simulink model "sampleModel1888"  (R2023a)
settings: Solver=VariableStepAuto  StartTime=0.0  StopTime=10.0  RelTol=1e-3
libraries: hdlsllib x4, simulink x3
settings Model: Creator=user1  LastModifiedBy=user1

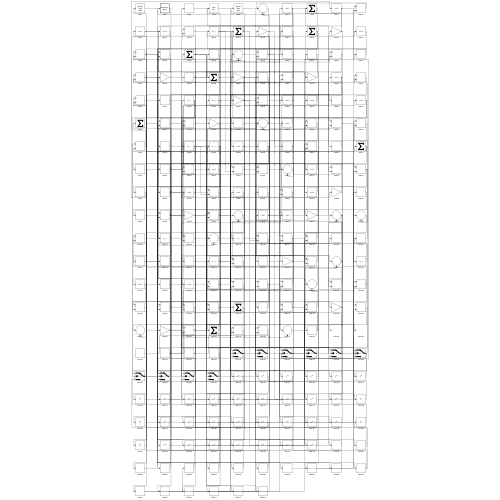
[thumbnail: Simulink's stored preview of the top-level diagram]
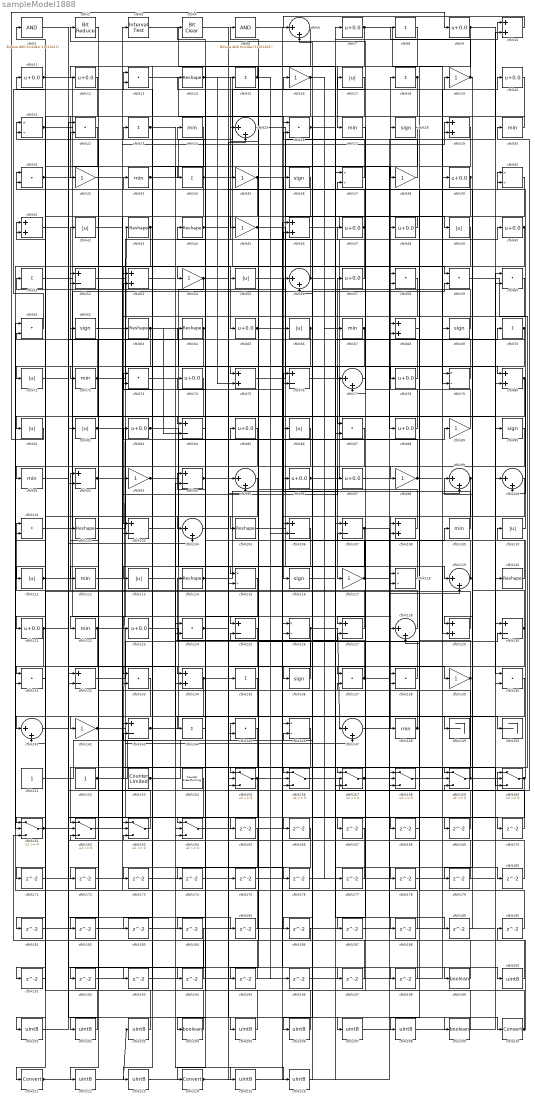
== system sampleModel1888 ==
  cfblk1 : simulink/Logic and Bit Operations/Bitwise Operator  logicop=AND  UseBitMask=on  BitMask=bin2dec('11011001')  BitMaskRealWorld=Stored Integer
      settings: LibrarySourceBlock=|
      | hdlsllib/Logic and Bit
      | Operations/Bitwise
      | Operator
  cfblk{10,29,41,46,53,68,75,80,108,129,134} (11 alike) : Sum
  cfblk{6,25,56,77,95,99..100,104,119,128,141,147} (12 alike) : Sum  Inputs=|++
  cfblk{13,22,26,31,58..61,73,87,101,124,131,133,137..138,140,145} (18 alike) : DotProduct  OutDataTypeStr=Inherit: Inherit via internal rule
  cfblk{14,43..44,63..64,102,105,114,120} (9 alike) : Reshape
  cfblk{52,76,84,92,94,103,106..107,125,127,130,132,143} (13 alike) : Sum  Inputs=+-
  cfblk{24,27,30,33,67,72,91,109,112,122,148} (11 alike) : MinMax
  cfblk{7,9,11..12,20,39,47..48,50,57,65,74,78,83,85,88,96..97,121,123} (20 alike) : Bias  Bias=0.0  SaturateOnIntegerOverflow=off
  cfblk{17,42,49,55,66,71,81..82,86,110..111,113} (12 alike) : Abs  SaturateOnIntegerOverflow=off
  cfblk{21,37,40,79,115,118,126,146} (8 alike) : Product  Inputs=*/  RndMeth=Zero  SaturateOnIntegerOverflow=on
  cfblk{28,36,62,69,90,116,136} (7 alike) : Signum
  cfblk{16,19,32,35,38,45,54,89,93,98,117,139,142} (13 alike) : Gain
  cfblk{8,15,18,23,34,51,70,135,144} (9 alike) : Sum  Inputs=+
  cfblk149 : Terminator
  cfblk150 : Terminator
  cfblk151 : Constant  SampleTime=-1
  cfblk152 : Constant  SampleTime=-1
  cfblk153 : hdlsllib/Sources/Counter Limited  uplimit=7  tsamp=-1
  cfblk154 : hdlsllib/Sources/Counter Free-Running  NumBits=16  tsamp=-1
  cfblk{155..164} (10 alike) : Switch  SaturateOnIntegerOverflow=off  InputSameDT=off
  cfblk{165..198} (34 alike) : Delay  SampleTime=1
  cfblk199 : DataTypeConversion  OutDataTypeStr=boolean  SaturateOnIntegerOverflow=off  RndMeth=Floor
  cfblk2 : hdlsllib/Logic and Bit Operations/Bit Reduce  mode=AND
  cfblk{200..203,205..208,212..213,215..216} (12 alike) : DataTypeConversion  OutDataTypeStr=uint8  SaturateOnIntegerOverflow=off  RndMeth=Floor
  cfblk204 : DataTypeConversion  OutDataTypeStr=boolean  SaturateOnIntegerOverflow=off  RndMeth=Floor
  cfblk209 : DataTypeConversion  OutDataTypeStr=boolean  SaturateOnIntegerOverflow=off  RndMeth=Floor
  cfblk210 : DataTypeConversion  SaturateOnIntegerOverflow=off  RndMeth=Floor
  cfblk211 : DataTypeConversion  SaturateOnIntegerOverflow=off  RndMeth=Floor
  cfblk214 : DataTypeConversion  SaturateOnIntegerOverflow=off  RndMeth=Floor
  cfblk3 : hdlsllib/Logic and Bit Operations/Interval Test  IntervalClosedRight=on  uplimit=0.5  IntervalClosedLeft=on  lowlimit=-0.5  OutDataTypeStr=boolean
  cfblk4 : simulink/Logic and Bit Operations/Bit Clear  iBit=0
      settings: LibrarySourceBlock=|
      | hdlsllib/Logic and Bit
      | Operations/Bit Clear
  cfblk5 : simulink/Logic and Bit Operations/Bitwise Operator  logicop=AND  UseBitMask=on  BitMask=bin2dec('11011001')  BitMaskRealWorld=Stored Integer
      settings: LibrarySourceBlock=|
      | hdlsllib/Logic and Bit
      | Operations/Bitwise
      | Operator
  wires:
  cfblk122/1 -> cfblk164/1, cfblk131/1
  cfblk75/1 -> cfblk40/1
  cfblk153/1 -> cfblk51/1, cfblk86/1
  cfblk80/1 -> cfblk100/2, cfblk212/1
  cfblk70/1 -> cfblk61/2, cfblk187/1
  cfblk59/1 -> cfblk156/1
  cfblk160/1 -> cfblk110/1, cfblk186/1
  cfblk14/1 -> cfblk59/1, cfblk75/2, cfblk159/2
  cfblk99/1 -> cfblk148/1, cfblk149/1
  cfblk31/1 -> cfblk65/1, cfblk133/2
  cfblk46/1 -> cfblk49/1
  cfblk21/1 -> cfblk125/1, cfblk193/1
  cfblk118/1 -> cfblk24/1
  cfblk132/1 -> cfblk130/2
  cfblk16/1 -> cfblk54/1, cfblk67/1
  cfblk13/1 -> cfblk116/1
  cfblk88/1 -> cfblk18/1
  cfblk155/1 -> cfblk109/1, cfblk183/1
  cfblk152/1 -> cfblk43/1, cfblk94/2
  cfblk146/1 -> cfblk214/1
  cfblk102/1 -> cfblk39/1
  cfblk161/1 -> cfblk160/1, cfblk185/1
  cfblk8/1 -> cfblk27/1
  cfblk19/1 -> cfblk129/1, cfblk8/1
  cfblk45/1 -> cfblk118/1, cfblk106/2
  cfblk143/1 -> cfblk47/1, cfblk127/2
  cfblk136/1 -> cfblk114/1
  cfblk164/1 -> cfblk46/1
  cfblk57/1 -> cfblk55/1
  cfblk79/1 -> cfblk42/1
  cfblk90/1 -> cfblk117/1
  cfblk63/1 -> cfblk75/1, cfblk72/1, cfblk84/2, cfblk160/3
  cfblk96/1 -> cfblk50/1, cfblk46/2, cfblk70/1
  cfblk159/1 -> cfblk90/1, cfblk137/2
  cfblk109/1 -> cfblk76/1
  cfblk82/1 -> cfblk128/1, cfblk29/2, cfblk134/2
  cfblk26/1 -> cfblk177/1, cfblk178/1
  cfblk72/1 -> cfblk15/1, cfblk77/1, cfblk41/2, cfblk111/1
  cfblk55/1 -> cfblk78/1
  cfblk74/1 -> cfblk81/1
  cfblk101/1 -> cfblk58/1
  cfblk113/1 -> cfblk157/1
  cfblk9/1 -> cfblk140/1, cfblk208/1
  cfblk43/1 -> cfblk103/1, cfblk103/2, cfblk131/2
  cfblk156/1 -> cfblk30/1
  cfblk85/1 -> cfblk93/1
  cfblk17/1 -> cfblk136/1
  cfblk97/1 -> cfblk68/1
  cfblk145/1 -> cfblk162/1
  cfblk83/1 -> cfblk118/2, cfblk23/1
  cfblk111/1 -> cfblk123/1, cfblk104/2
  cfblk18/1 -> cfblk32/1, cfblk121/1
  cfblk61/1 -> cfblk13/1
  cfblk87/1 -> cfblk91/1
  cfblk69/1 -> cfblk14/1
  cfblk36/1 -> cfblk122/1
  cfblk123/1 -> cfblk125/2
  cfblk58/1 -> cfblk113/1
  cfblk73/1 -> cfblk56/1
  cfblk114/1 -> cfblk57/1, cfblk139/1
  cfblk29/1 -> cfblk98/1
  cfblk54/1 -> cfblk53/2, cfblk170/1
  cfblk86/1 -> cfblk115/1
  cfblk56/1 -> cfblk10/1, cfblk35/1
  cfblk3/1 -> cfblk107/1
  cfblk128/1 -> cfblk101/1
  cfblk51/1 -> cfblk87/1
  cfblk124/1 -> cfblk44/1, cfblk37/2, cfblk194/1
  cfblk66/1 -> cfblk126/2, cfblk191/1
  cfblk89/1 -> cfblk2/1
  cfblk48/1 -> cfblk45/1
  cfblk120/1 -> cfblk74/1
  cfblk81/1 -> cfblk9/1
  cfblk110/1 -> cfblk40/2
  cfblk117/1 -> cfblk48/1, cfblk36/1
  cfblk154/1 -> cfblk162/2
  cfblk93/1 -> cfblk89/1, cfblk159/1
  cfblk44/1 -> cfblk134/1, cfblk166/1
  cfblk126/1 -> cfblk147/1, cfblk171/1
  cfblk33/1 -> cfblk19/1, cfblk38/1
  cfblk121/1 -> cfblk64/1, cfblk161/2
  cfblk112/1 -> cfblk155/1
  cfblk95/1 -> cfblk211/1
  cfblk30/1 -> cfblk26/1
  cfblk84/1 -> cfblk144/1
  cfblk127/1 -> cfblk92/1
  cfblk158/1 -> cfblk99/2
  cfblk139/1 -> cfblk31/1, cfblk156/3
  cfblk142/1 -> cfblk147/2, cfblk168/1
  cfblk140/1 -> cfblk143/1
  cfblk40/1 -> cfblk155/2
  cfblk28/1 -> cfblk156/2
  cfblk32/1 -> cfblk3/1
  cfblk77/1 -> cfblk127/1
  cfblk50/1 -> cfblk141/1, cfblk77/2
  cfblk98/1 -> cfblk20/1, cfblk13/2
  cfblk67/1 -> cfblk161/1, cfblk17/1
  cfblk92/1 -> cfblk76/2, cfblk164/3, cfblk160/2
  cfblk42/1 -> cfblk80/1
  cfblk108/1 -> cfblk25/1
  cfblk38/1 -> cfblk28/1
  cfblk49/1 -> cfblk104/1
  cfblk131/1 -> cfblk141/2
  cfblk137/1 -> cfblk96/1, cfblk189/1
  cfblk35/1 -> cfblk10/2, cfblk71/1, cfblk197/1
  cfblk27/1 -> cfblk137/1
  cfblk148/1 -> cfblk73/1, cfblk102/1
  cfblk135/1 -> cfblk164/2
  cfblk37/1 -> cfblk16/1
  cfblk68/1 -> cfblk108/1
  cfblk39/1 -> cfblk112/1, cfblk124/2
  cfblk78/1 -> cfblk41/1
  cfblk100/1 -> cfblk106/1
  cfblk20/1 -> cfblk132/2
  cfblk157/1 -> cfblk29/1, cfblk119/2
  cfblk10/1 -> cfblk6/1
  cfblk34/1 -> cfblk163/2, cfblk7/1, cfblk21/2
  cfblk163/1 -> cfblk52/1
  cfblk151/1 -> cfblk145/1
  cfblk25/1 -> cfblk79/2
  cfblk4/1 -> cfblk210/1
  cfblk7/1 -> cfblk69/1, cfblk63/1, cfblk195/1
  cfblk47/1 -> cfblk145/2, cfblk33/1
  cfblk129/1 -> cfblk21/1
  cfblk64/1 -> cfblk84/1, cfblk182/1, cfblk184/1
  cfblk62/1 -> cfblk120/1
  cfblk105/1 -> cfblk129/2
  cfblk130/1 -> cfblk158/2, cfblk31/2
  cfblk12/1 -> cfblk92/2
  cfblk119/1 -> cfblk26/2, cfblk179/1
  cfblk15/1 -> cfblk12/1, cfblk196/1
  cfblk134/1 -> cfblk142/1, cfblk167/1
  cfblk103/1 -> cfblk150/1
  cfblk94/1 -> cfblk155/3, cfblk59/2
  cfblk162/1 -> cfblk97/1
  cfblk76/1 -> cfblk100/1
  cfblk11/1 -> cfblk135/1, cfblk88/1
  cfblk52/1 -> cfblk124/1
  cfblk138/1 -> cfblk85/1
  cfblk144/1 -> cfblk94/1
  cfblk23/1 -> cfblk119/1, cfblk176/1, cfblk199/1
  cfblk106/1 -> cfblk115/2
  cfblk6/1 -> cfblk34/1
  cfblk65/1 -> cfblk66/1, cfblk105/1
  cfblk107/1 -> cfblk133/1, cfblk180/1
  cfblk91/1 -> cfblk165/1
  cfblk167/1 -> cfblk163/3
  cfblk168/1 -> cfblk68/2
  cfblk147/1 -> cfblk169/1
  cfblk169/1 -> cfblk157/2
  cfblk170/1 -> cfblk99/1
  cfblk171/1 -> cfblk158/3
  cfblk2/1 -> cfblk172/1
  cfblk172/1 -> cfblk53/1
  cfblk24/1 -> cfblk173/1
  cfblk115/1 -> cfblk174/1
  cfblk174/1 -> cfblk25/2
  cfblk104/1 -> cfblk175/1
  cfblk175/1 -> cfblk157/3
  cfblk176/1 -> cfblk138/1
  cfblk177/1 -> cfblk132/1
  cfblk178/1 -> cfblk80/2
  cfblk179/1 -> cfblk56/2
  cfblk180/1 -> cfblk6/2
  cfblk133/1 -> cfblk181/1
  cfblk181/1 -> cfblk37/1
  cfblk182/1 -> cfblk52/2
  cfblk183/1 -> cfblk140/2
  cfblk185/1 -> cfblk163/1
  cfblk186/1 -> cfblk161/3
  cfblk187/1 -> cfblk130/1
  cfblk116/1 -> cfblk188/1
  cfblk188/1 -> cfblk61/1
  cfblk189/1 -> cfblk159/3
  cfblk190/1 -> cfblk128/2
  cfblk191/1 -> cfblk101/2
  cfblk125/1 -> cfblk192/1
  cfblk192/1 -> cfblk79/1
  cfblk193/1 -> cfblk108/2
  cfblk194/1 -> cfblk143/2
  cfblk195/1 -> cfblk73/2
  cfblk196/1 -> cfblk58/2
  cfblk197/1 -> cfblk162/3
  cfblk71/1 -> cfblk198/1
  cfblk198/1 -> cfblk158/1
  cfblk199/1 -> cfblk5/1
  cfblk5/1 -> cfblk200/1
  cfblk200/1 -> cfblk11/1
  cfblk22/1 -> cfblk201/1
  cfblk201/1 -> cfblk82/1
  cfblk184/1 -> cfblk202/1
  cfblk202/1 -> cfblk22/1
  cfblk203/1 -> cfblk22/2
  cfblk166/1 -> cfblk204/1
  cfblk204/1 -> cfblk1/1
  cfblk1/1 -> cfblk205/1
  cfblk205/1 -> cfblk62/1
  cfblk60/1 -> cfblk206/1
  cfblk206/1 -> cfblk83/1
  cfblk141/1 -> cfblk207/1
  cfblk207/1 -> cfblk60/1
  cfblk208/1 -> cfblk60/2
  cfblk41/1 -> cfblk209/1
  cfblk209/1 -> cfblk4/1
  cfblk210/1 -> cfblk190/1, cfblk107/2
  cfblk211/1 -> cfblk203/1, cfblk87/2
  cfblk212/1 -> cfblk95/1
  cfblk165/1 -> cfblk213/1
  cfblk213/1 -> cfblk95/2
  cfblk214/1 -> cfblk138/2, cfblk126/1
  cfblk173/1 -> cfblk215/1
  cfblk215/1 -> cfblk146/1
  cfblk53/1 -> cfblk216/1
  cfblk216/1 -> cfblk146/2
